simulink model "flow"  (R2018a)
settings: Solver=FixedStepDiscrete  StartTime=0.0  StopTime=10  FixedStep=0.1  RelTol=1e-3  EnableMultiTasking=on
settings Model: Creator=lenovo  LastModifiedBy=DELL
settings SolverCC: AutoInsertRateTranBlk=on
settings DataIOCC: LimitDataPoints=on
settings OptimizationCC: LifeSpan=inf
settings DebuggingCC: AllowSymbolicDim=off  SFUnexpectedBacktrackingDiag=warning  SFNoUnconditionalDefaultTransitionDiag=warning  SFExecutionAtInitializationDiag=none
settings CodeAppCC: StateflowObjectComments=on
settings GRTTargetCC: TargetLangStandard=C89/C90 (ANSI)
settings ConfigComp: CovMetricSettings=dw  CovHtmlReporting=on  CovSaveCumulativeToWorkspaceVar=on  CovSaveSingleToWorkspaceVar=on  CovShowResultsExplorer=off  CovExternalEMLEnable=off  CovSFcnEnable=off

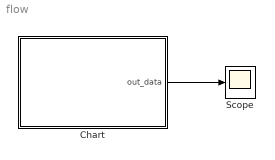
== system flow ==
  Chart : Stateflow chart  TreatAsAtomicUnit=on
  Scope : Scope
  wires:
  Chart/1(out_data) -> Scope/1

== stateflow chart flow/Chart ==
  state A
  state B
    (default) -> (junction 10) : {i=1;}
    (junction 10) -> (junction 12) [order 1] : [i<=3]
    (junction 13) -> (junction 10) : {i = i + 1;}
    (junction 10) -> (junction 14) [order 2]
    (junction 12) -> (junction 13) : {out_data(i)=out_data(i)+i;}
  (default) -> A
  A -> B
  B -> A
  data: out_data output =[0,0,0]; i local
